simulink model "multadd_flex_tb1"  (R2019b)
settings: Solver=FixedStepDiscrete  StartTime=0.0  StopTime=1000  RelTol=1e-3
libraries: lib_dsphdlmath_v1 x6, simulink x2, dspsrcs4 x1
settings Model: DataTypeOverride=Off  Creator=mbabst  LastModifiedBy=mbabst
settings DataIOCC: SaveOutput=off  SaveTime=off  ReturnWorkspaceOutputs=off
settings OptimizationCC: BlockReduction=off  ConditionallyExecuteInputs=off  DefaultParameterBehavior=Inlined  LifeSpan=inf
settings DebuggingCC: AlgebraicLoopMsg=error  SingleTaskRateTransMsg=error  StrictBusMsg=ErrorOnBusTreatedAsVector  SFUnexpectedBacktrackingDiag=warning  SFNoUnconditionalDefaultTransitionDiag=warning  SFExecutionAtInitializationDiag=none  ArithmeticOperatorsInVariantConditions=warning
settings HardwareCC: ProdBitPerPointer=32  ProdBitPerSizeT=32  ProdBitPerPtrDiffT=32  ProdLargestAtomicFloat=None  ProdIntDivRoundTo=Undefined  ProdEndianess=Unspecified  ProdWordSize=32  ProdHWDeviceType=ASIC/FPGA->ASIC/FPGA  ProdEqTarget=off
settings SFSimCC: SimUseLocalCustomCode=off  CustomCodeUndefinedFunction=UseInterfaceOnly
settings RTWCC: RTWUseLocalCustomCode=off
settings CodeAppCC: StateflowObjectComments=on
settings GRTTargetCC: TargetLangStandard=C89/C90 (ANSI)
settings ConfigComp: CovMetricSettings=dw  CovHtmlReporting=on  CovSaveCumulativeToWorkspaceVar=on  CovSaveSingleToWorkspaceVar=on  CovExternalEMLEnable=off

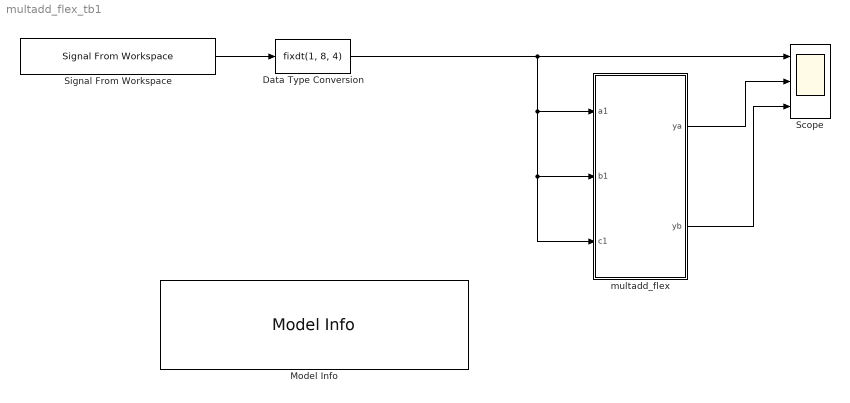
== system multadd_flex_tb1 ==
  Data Type Conversion : DataTypeConversion  OutDataTypeStr=fixdt(1, 8, 4)  ConvertRealWorld=Stored Integer (SI)
  Model Info : simulink/Model-Wide Utilities/Model Info  Frame=on  DisplayStringWithTags=|  HorizontalTextAlignment=Left  LeftAlignmentValue=0.02
      | Copyright (c) 2005-2021 DSPlogic, Inc.
      | Distributed under the terms of the Simplified BSD License.
      | The full license is in the file LICENSE, distributed with this software.
      | 
      | Model: %<ModelName> (v%<ModelVersion>)
      | Author: Michael Babst <mike.babst@dsplogic.com>
      | Created: by %<Creator> on %<Created>
      | Modified: by %<ModifiedBy> on %<LastModificationDate>
  Scope : Scope  NumInputPorts=3
  Signal From Workspace : dspsrcs4/Signal From Workspace  X=[(0:2^7-1) (2^7-1-2:-1:-2^7 ) (-2^7 : -1) ]  Ts=1  nsamps=1  OutputAfterFinalValue=Cyclic repetition  ignoreOrWarnInputAndFrameLengths=on  OutputFrames=off
  multadd_flex : Subsystem
  wires:
  multadd_flex/1(ya) -> Scope/2
  multadd_flex/2(yb) -> Scope/3
  Signal From Workspace/1 -> Data Type Conversion/1
  Data Type Conversion/1 -> multadd_flex/2(b1), multadd_flex/3(c1), multadd_flex/1(a1), Scope/1

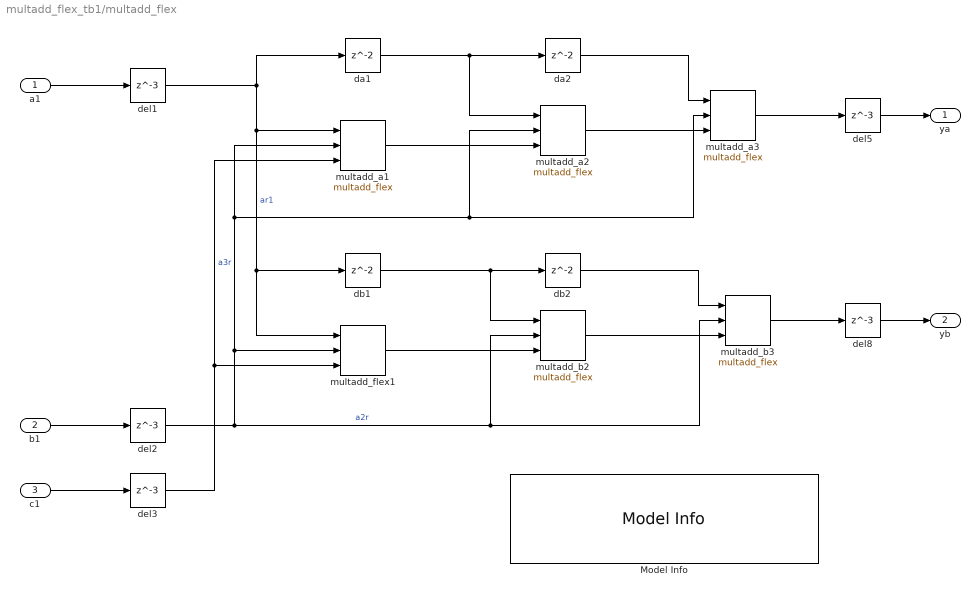
== system multadd_flex_tb1/multadd_flex ==
  a1 : Inport
  b1 : Inport  Port=2
  c1 : Inport  Port=3
  Model Info : simulink/Model-Wide Utilities/Model Info  Frame=on  DisplayStringWithTags=|  HorizontalTextAlignment=Left  LeftAlignmentValue=0.02
      | Copyright (c) 2005-2021 DSPlogic, Inc.
      | Distributed under the terms of the Simplified BSD License.
      | The full license is in the file LICENSE, distributed with this software.
      | 
      | Model: %<ModelName> (v%<ModelVersion>)
      | Author: Michael Babst <mike.babst@dsplogic.com>
      | Created: by %<Creator> on %<Created>
      | Modified: by %<ModifiedBy> on %<LastModificationDate>
  da1 : Delay  InitialCondition=0
  da2 : Delay  InitialCondition=0
  db1 : Delay  InitialCondition=0
  db2 : Delay  InitialCondition=0
  del{1..3,5,8} (5 alike) : Delay  DelayLength=3  InitialCondition=0
  multadd_a1 : lib_dsphdlmath_v1/multadd_flex  accumMode=Automatic  Nd_in=1  Nd_out=1  Wa=18  extend_a=off  scalingSelect_a=Best Precision  Sforce_a=0  roundMode_a=Floor  saturate_a=off  Wb=18  extend_b=off  scalingSelect_b=Best Precision  Sforce_b=0  roundMode_b=Floor  saturate_b=off  Wc=63  extend_c=off  scalingSelect_c=Best Range  Sforce_c=0  roundMode_c=Floor  saturate_c=off
      settings: SourceProductName=DSPHDL Library
  multadd_a2 : lib_dsphdlmath_v1/multadd_flex  accumMode=Automatic  Nd_in=1  Nd_out=1  Wa=18  extend_a=off  scalingSelect_a=Best Precision  Sforce_a=0  roundMode_a=Floor  saturate_a=off  Wb=18  extend_b=off  scalingSelect_b=Best Precision  Sforce_b=0  roundMode_b=Floor  saturate_b=off  Wc=63  extend_c=off  scalingSelect_c=Best Range  Sforce_c=0  roundMode_c=Floor  saturate_c=off
      settings: SourceProductName=DSPHDL Library
  multadd_a3 : lib_dsphdlmath_v1/multadd_flex  accumMode=Automatic  Nd_in=1  Nd_out=1  Wa=18  extend_a=off  scalingSelect_a=Best Precision  Sforce_a=0  roundMode_a=Floor  saturate_a=off  Wb=18  extend_b=off  scalingSelect_b=Best Precision  Sforce_b=0  roundMode_b=Floor  saturate_b=off  Wc=63  extend_c=off  scalingSelect_c=Best Range  Sforce_c=0  roundMode_c=Floor  saturate_c=off
      settings: SourceProductName=DSPHDL Library
  multadd_b2 : lib_dsphdlmath_v1/multadd_flex  accumMode=Automatic  Nd_in=1  Nd_out=1  Wa=18  extend_a=on  scalingSelect_a=Best Precision  Sforce_a=0  roundMode_a=Floor  saturate_a=off  Wb=18  extend_b=on  scalingSelect_b=Best Precision  Sforce_b=0  roundMode_b=Floor  saturate_b=off  Wc=63  extend_c=off  scalingSelect_c=Best Range  Sforce_c=0  roundMode_c=Floor  saturate_c=off
      settings: SourceProductName=DSPHDL Library
  multadd_b3 : lib_dsphdlmath_v1/multadd_flex  accumMode=Automatic  Nd_in=1  Nd_out=1  Wa=18  extend_a=on  scalingSelect_a=Best Precision  Sforce_a=0  roundMode_a=Floor  saturate_a=off  Wb=18  extend_b=on  scalingSelect_b=Best Precision  Sforce_b=0  roundMode_b=Floor  saturate_b=off  Wc=63  extend_c=off  scalingSelect_c=Best Range  Sforce_c=0  roundMode_c=Floor  saturate_c=off
      settings: SourceProductName=DSPHDL Library
  multadd_flex1 : lib_dsphdlmath_v1/multadd_flex  accumMode=Automatic  Nd_in=1  Nd_out=1  Wa=18  extend_a=on  scalingSelect_a=Best Precision  Sforce_a=0  roundMode_a=Floor  saturate_a=off  Wb=18  extend_b=on  scalingSelect_b=Best Precision  Sforce_b=0  roundMode_b=Floor  saturate_b=off  Wc=63  extend_c=off  scalingSelect_c=Best Precision  Sforce_c=60  roundMode_c=Floor  saturate_c=off
      settings: SourceProductName=DSPHDL Library
  ya : Outport
  yb : Outport  Port=2
  wires:
  a1/1 -> del1/1
  b1/1 -> del2/1
  c1/1 -> del3/1
  del1/1 -> multadd_flex1/1, db1/1, multadd_a1/1, da1/1  "ar1"
  del2/1 -> multadd_b2/2, multadd_b3/2, multadd_flex1/2, multadd_a2/2, multadd_a3/2, multadd_a1/2  "a2r"
  del3/1 -> multadd_flex1/3, multadd_a1/3  "a3r"
  multadd_a1/1 -> multadd_a2/3
  multadd_a2/1 -> multadd_a3/3
  del5/1 -> ya/1
  multadd_flex1/1 -> multadd_b2/3
  multadd_b2/1 -> multadd_b3/3
  multadd_b3/1 -> del8/1
  del8/1 -> yb/1
  multadd_a3/1 -> del5/1
  db1/1 -> multadd_b2/1, db2/1
  db2/1 -> multadd_b3/1
  da2/1 -> multadd_a3/1
  da1/1 -> multadd_a2/1, da2/1
